simulink model "m005_SimulEqn"  (R2022a)
settings: Solver=VariableStepAuto  StartTime=0.0  StopTime=10.0  RelTol=1e-3
settings Model: Creator=Admin  LastModifiedBy=Admin

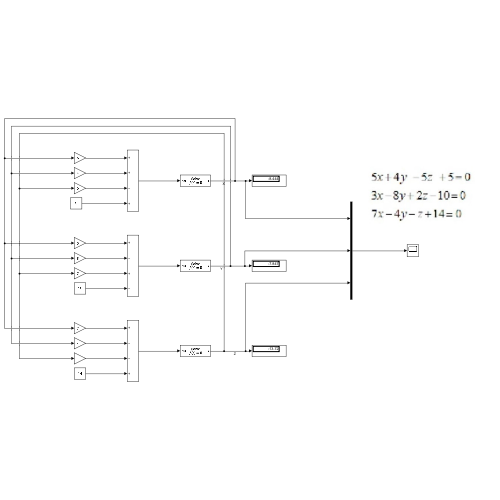
[thumbnail: Simulink's stored preview of the top-level diagram]
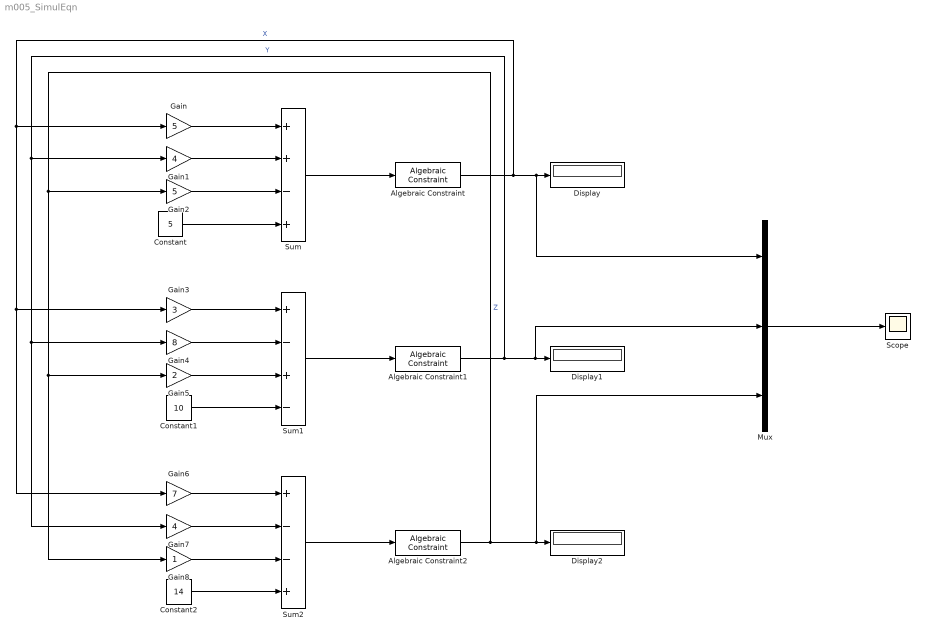
== system m005_SimulEqn ==
  Algebraic Constraint : AlgebraicConstraint
  Algebraic Constraint1 : AlgebraicConstraint
  Algebraic Constraint2 : AlgebraicConstraint
  Constant : Constant  Value=5
  Constant1 : Constant  Value=10
  Constant2 : Constant  Value=14
  Display : Display
  Display1 : Display
  Display2 : Display
  Gain : Gain  Gain=5
  Gain1 : Gain  Gain=4
  Gain2 : Gain  Gain=5
  Gain3 : Gain  Gain=3
  Gain4 : Gain  Gain=8
  Gain5 : Gain  Gain=2
  Gain6 : Gain  Gain=7
  Gain7 : Gain  Gain=4
  Gain8 : Gain
  Mux : Mux  Inputs=3
  Scope : Scope
  Sum : Sum  Inputs=++-+
  Sum1 : Sum  Inputs=+-+-
  Sum2 : Sum  Inputs=+--+
  wires:
  Algebraic Constraint/1 -> Gain6/1, Gain3/1, Gain/1, Mux/1, Display/1  "X"
  Algebraic Constraint1/1 -> Gain7/1, Gain4/1, Gain1/1, Mux/2, Display1/1  "Y"
  Algebraic Constraint2/1 -> Gain8/1, Gain5/1, Gain2/1, Mux/3, Display2/1  "Z"
  Sum/1 -> Algebraic Constraint/1
  Sum1/1 -> Algebraic Constraint1/1
  Sum2/1 -> Algebraic Constraint2/1
  Gain/1 -> Sum/1
  Gain1/1 -> Sum/2
  Gain2/1 -> Sum/3
  Constant/1 -> Sum/4
  Gain3/1 -> Sum1/1
  Gain4/1 -> Sum1/2
  Gain5/1 -> Sum1/3
  Constant1/1 -> Sum1/4
  Gain6/1 -> Sum2/1
  Gain7/1 -> Sum2/2
  Gain8/1 -> Sum2/3
  Constant2/1 -> Sum2/4
  Mux/1 -> Scope/1
